simulink model "Path_following_Model_w_dbl_lane_change"  (R2018a)
settings: Solver=VariableStepAuto  StartTime=0.0  StopTime=inf  FixedStep=1  RelTol=1e-3
values from neighbouring files (symbols this model uses):
  A_matrix = [a11 a12 0 0; a21 a22 0 0; 0 1 0 0; V ls V 0]    [Path_following_SS.m]
  B_matrix = [b11 0; b21 0; 0 -V; 0 -ls*V]    [Path_following_SS.m]
  C_matrix = [1 0 0 0; 0 1 0 0; 0 0 1 0; 0 0 0 1]    [Path_following_SS.m]
  D_matrix = [0 0; 0 0; 0 0; 0 0]    [Path_following_SS.m]
  dis_vec = Cum_dis(1:end-1)    [Double_lane_change_bezier_func_mcode_V2.m]
  rho_new = (((del_1_Xp(2:end)/del_pts).*(del_2_Yp/del_pts.^2))-((del_1_Yp(2:end)/del_pts).*((del_2_Xp/del_pts.^2))))./((del_1_Xp(2:end)./del_pts).^2+((del_1_Yp(2:end)./del_pts).^2)).^1.5    [Double_lane_change_bezier_func_mcode_V2.m]
  V = 5    [Path_following_SS.m]
  Xp = [Xp_1(1:end-1); Xp_2(1:end-1); Xp_3(1:end-1);]    [Double_lane_change_bezier_func_mcode_V2.m]
  Yp = [Yp_1(1:end-1); Yp_2(1:end-1); Yp_3(1:end-1);]    [Double_lane_change_bezier_func_mcode_V2.m]
undefined symbols (not defined in the file or in its folder): Cum_dis, sigbuilder_block
libraries: simulink x2
settings Model: Creator=Santo  LastModifiedBy=SYG

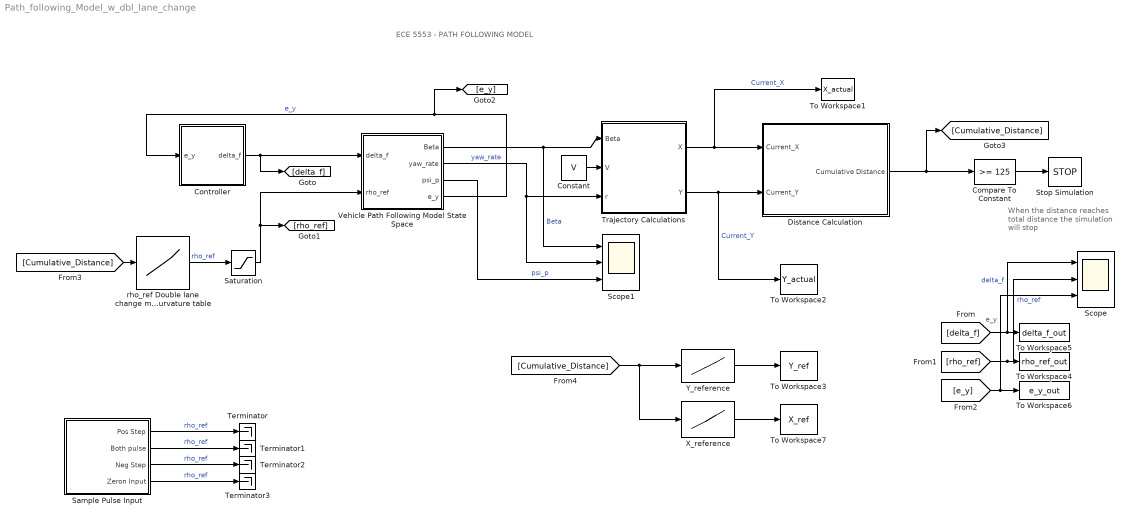
== system Path_following_Model_w_dbl_lane_change ==
  note: When the distance reaches total distance the simulation will stop
  note: ECE 5553 - PATH FOLLOWING MODEL
  Compare To Constant : simulink/Logic and Bit Operations/Compare To Constant  relop=>=  const=125  OutDataTypeStr=boolean
  Constant : Constant  Value=V
  Controller : Subsystem
  Distance Calculation : Subsystem
  Sample Pulse Input : Subsystem  Tag=STV Subsys  LoadFcn=sigbuilder_block('load');  StartFcn=sigbuilder_block('start');  StopFcn=sigbuilder_block('stop');  ClipboardFcn=sigbuilder_block('clipboard');  mask(Sigbuilder block){tuvar=[0:10]}
      mask help: Simulink:masks:SigbuilderBlock_MD
      mask init:
      | if ~strcmp(get_param(bdroot(gcbh),'SimulationStatus'),'stopped') tuvar = sigbuilder_block('maskInit'); end
      settings: CopyFcn=sigbuilder_block('copy');  DeleteFcn=sigbuilder_block('delete');  ModelCloseFcn=sigbuilder_block('modelClose');  PreSaveFcn=sigbuilder_block('preSave');  PauseFcn=sigbuilder_block('pause');  ContinueFcn=sigbuilder_block('continue');  NameChangeFcn=sigbuilder_block('namechange');  OpenFcn=sigbuilder_block('open',[6 24 1012.5 453.75 ]);  CloseFcn=sigbuilder_block('close');
      mask Display: plot(0, 0, 100, 100,[2, 2, 32, 32, 2], [68, 8, 8, 68, 68],[32, 2], [38, 38], [32, 19, 2],[53, 60, 44], [32, 17, 17, 2],[16, 16, 31, 31]);txt = getActiveGroup(gcbh);text(2, 100, txt,'verticalAlignment', 'top');
  Saturation : Saturate  UpperLimit=0.01  LowerLimit=-0.025  LinearizeAsGain=off
  Scope : Scope  NumInputPorts=3
  Scope1 : Scope  NumInputPorts=3
  Stop Simulation : Stop
  Terminator{,1..3} (4 alike) : Terminator
  To Workspace1 : ToWorkspace  VariableName=X_actual  SampleTime=-1
  To Workspace2 : ToWorkspace  VariableName=Y_actual  SampleTime=-1
  To Workspace3 : ToWorkspace  VariableName=Y_ref  SampleTime=-1
  To Workspace4 : ToWorkspace  VariableName=rho_ref_out  SampleTime=-1
  To Workspace5 : ToWorkspace  VariableName=delta_f_out  SampleTime=-1
  To Workspace6 : ToWorkspace  VariableName=e_y_out  SampleTime=-1
  To Workspace7 : ToWorkspace  VariableName=X_ref  SampleTime=-1
  Trajectory Calculations : Subsystem
  Vehicle Path Following Model State Space : Subsystem
  X_reference : Lookup_n-D  NumberOfTableDimensions=1  BreakpointsForDimension1=Cum_dis  Table=Xp(1:end-1)  InternalRulePriority=Speed  RndMeth=Simplest  InputSameDT=on
  Y_reference : Lookup_n-D  NumberOfTableDimensions=1  BreakpointsForDimension1=Cum_dis  Table=Yp(1:end-1)  InternalRulePriority=Speed  RndMeth=Simplest  InputSameDT=on
  rho_ref Double lane change manoeuver distanced based Road curvature table : Lookup_n-D  NumberOfTableDimensions=1  BreakpointsForDimension1=dis_vec  Table=rho_new  InternalRulePriority=Speed  RndMeth=Simplest  InputSameDT=on
  wires:
  Trajectory Calculations/1(X) -> Distance Calculation/1(Current_X), To Workspace1/1  "Current_X"
  Constant/1 -> Trajectory Calculations/2(V)
  Vehicle Path Following Model State Space/4(e_y) -> [e_y], Controller/1(e_y)  "e_y"
  Vehicle Path Following Model State Space/1(Beta) -> Scope1/1, Trajectory Calculations/1(Beta)  "Beta"
  Vehicle Path Following Model State Space/2(yaw_rate) -> Scope1/2, Trajectory Calculations/3(r)  "yaw_rate"
  Controller/1(delta_f) -> [delta_f], Vehicle Path Following Model State Space/1(delta_f)
  [delta_f] -> Scope/1, To Workspace5/1  "delta_f"
  [rho_ref] -> Scope/2, To Workspace4/1  "rho_ref"
  [e_y] -> Scope/3, To Workspace6/1  "e_y"
  Vehicle Path Following Model State Space/3(psi_p) -> Scope1/3  "psi_p"
  Trajectory Calculations/2(Y) -> To Workspace2/1, Distance Calculation/2("Current_Y ")  "Current_Y"
  rho_ref Double lane change manoeuver distanced based Road curvature table/1 -> Saturation/1  "rho_ref"
  Compare To Constant/1 -> Stop Simulation/1
  Saturation/1 -> Vehicle Path Following Model State Space/2(rho_ref), [rho_ref]
  Distance Calculation/1(Cumulative Distance) -> [Cumulative_Distance], Compare To Constant/1
  Sample Pulse Input/1(Pos Step) -> Terminator/1  "rho_ref"
  Sample Pulse Input/2(Both pulse) -> Terminator1/1  "rho_ref"
  Sample Pulse Input/3(Neg Step) -> Terminator2/1  "rho_ref"
  Sample Pulse Input/4(Zeron Input) -> Terminator3/1  "rho_ref"
  X_reference/1 -> To Workspace7/1
  Y_reference/1 -> To Workspace3/1
  [Cumulative_Distance] -> rho_ref Double lane change manoeuver distanced based Road curvature table/1
  [Cumulative_Distance] -> X_reference/1, Y_reference/1

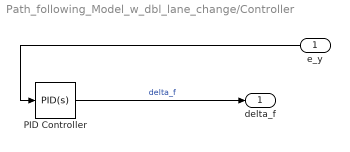
== system Path_following_Model_w_dbl_lane_change/Controller ==
  e_y : Inport
  PID Controller : simulink/Continuous/PID Controller  Controller=PID  TimeDomain=Continuous-time  SampleTime=-1  IntegratorMethod=Forward Euler  FilterMethod=Forward Euler  Form=Parallel  UseFilter=on  ControllerParametersSource=internal  P=-3.00951214129924  I=-3.08390402818753  D=0.0317765423784897  N=10.6234395055982  InitialConditionSource=internal  InitialConditionForIntegrator=0  InitialConditionForFilter=0  ExternalReset=none  LimitOutput=off  UpperSaturationLimit=inf  LowerSaturationLimit=-inf  LinearizeAsGain=on  AntiWindupMode=none  Kb=1  TrackingMode=off  Kt=1  PParamMin=[]  PParamMax=[]  IParamMin=[]  IParamMax=[]  DParamMin=[]  DParamMax=[]  NParamMin=[]  NParamMax=[]  KbParamMin=[]  KbParamMax=[]  KtParamMin=[]  KtParamMax=[]  POutMin=[]  POutMax=[]  IOutMin=[]  IOutMax=[]  DOutMin=[]  DOutMax=[]  NOutMin=[]  NOutMax=[]  KbOutMin=[]  KbOutMax=[]  KtOutMin=[]  KtOutMax=[]  IntegratorOutMin=[]  IntegratorOutMax=[]  FilterOutMin=[]  FilterOutMax=[]  SumOutMin=[]  SumOutMax=[]  SumI1OutMin=[]  SumI1OutMax=[]  SumI2OutMin=[]  SumI2OutMax=[]  SumI3OutMin=[]  SumI3OutMax=[]  SumDOutMin=[]  SumDOutMax=[]  SaturationOutMin=[]  SaturationOutMax=[]  IntegratorContinuousStateAttributes=''  IntegratorStateMustResolveToSignalObject=off  IntegratorRTWStateStorageClass=Auto  FilterContinuousStateAttributes=''  FilterStateMustResolveToSignalObject=off  FilterRTWStateStorageClass=Auto  DifferentiatorICPrevScaledInput=0  DifferentiatorOutMin=[]  DifferentiatorOutMax=[]  InitialConditionSetting=State (most efficient)  FilterDiffOutCoefMin=[]  FilterDiffOutCoefMax=[]  SumDenOutMin=[]  SumDenOutMax=[]  SumNumOutMin=[]  SumNumOutMax=[]  ReciprocalOutMin=[]  ReciprocalOutMax=[]  DivideOutMin=[]  DivideOutMax=[]  TunerSelectOption=Transfer Function Based (PID Tuner App)
  delta_f : Outport
  wires:
  PID Controller/1 -> delta_f/1  "delta_f"
  e_y/1 -> PID Controller/1

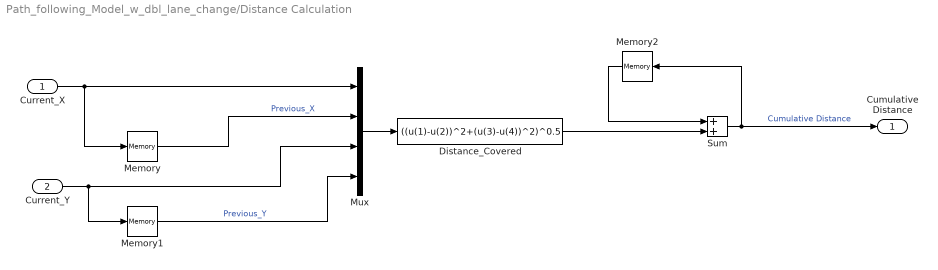
== system Path_following_Model_w_dbl_lane_change/Distance Calculation ==
  Current_X : Inport
  "Current_Y " : Inport  Port=2
  Distance_Covered : Fcn  Expr=((u(1)-u(2))^2+(u(3)-u(4))^2)^0.5
  Memory : Memory
  Memory1 : Memory
  Memory2 : Memory
  Mux : Mux
  Sum : Sum
  Cumulative Distance : Outport
  wires:
  Memory1/1 -> Mux/4  "Previous_Y"
  Mux/1 -> Distance_Covered/1
  Distance_Covered/1 -> Sum/2
  Memory/1 -> Mux/2  "Previous_X"
  Memory2/1 -> Sum/1
  "Current_Y "/1 -> Memory1/1, Mux/3
  Current_X/1 -> Memory/1, Mux/1
  Sum/1 -> Cumulative Distance/1, Memory2/1  "Cumulative Distance"

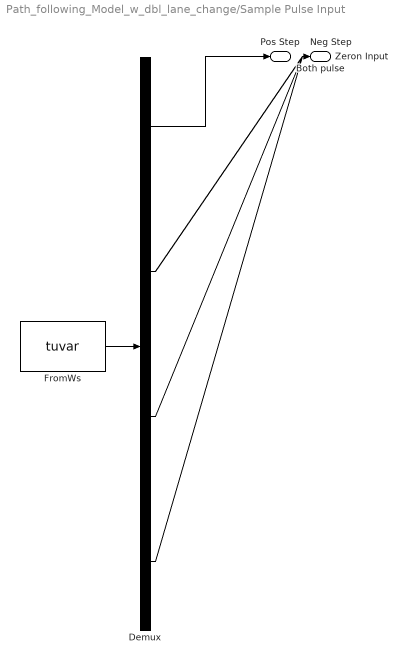
== system Path_following_Model_w_dbl_lane_change/Sample Pulse Input ==
  Demux : Demux  Tag=STV Demux
  FromWs : FromWorkspace  Tag=STV FromWs  VariableName=tuvar  SampleTime=0
      SigBuilderData=|
      | common.afterFinalStr = 'Extrapolate'
      | common.sampleTime = 0
      | dataSet.timeRange = [0 10]
      | dataSet.name = 'Group 1'
      | sbobj.Groups.Name = 'Group 1'
      | sbobj.Groups.Signals(1).Name = 'Pos Step'
      | sbobj.Groups.Signals(1).XData = [0 4 4 6 6 10]
      | sbobj.Groups.Signals(1).YData = [0 0 0.1 0.1 0 0]
      | sbobj.Groups.Signals(2).Name = 'Both pulse'
      | sbobj.Groups.Signals(2).XData = [0 4 4 6 6 7 7 9 9 10]
      | sbobj.Groups.Signals(2).YData = [0 0 0.1 0.1 0 0 -0.1 -0.1 0 0]
      | sbobj.Groups.Signals(3).Name = 'Neg Step'
      | sbobj.Groups.Signals(3).XData = [0 4 4 6 6 10]
      | sbobj.Groups.Signals(3).YData = [0 0 -0.1 -0.1 0 0]
      | sbobj.Groups.Signals(4).Name = 'Zeron Input'
      | sbobj.Groups.Signals(4).XData = [0 10]
      | sbobj.Groups.Signals(4).YData = [0 0]
  Pos Step : Outport  Tag=STV Outport
  Both pulse : Outport  Tag=STV Outport  Port=2
  Neg Step : Outport  Tag=STV Outport  Port=3
  Zeron Input : Outport  Tag=STV Outport  Port=4
  wires:
  FromWs/1 -> Demux/1
  Demux/1 -> Pos Step/1
  Demux/2 -> Both pulse/1
  Demux/3 -> Neg Step/1
  Demux/4 -> Zeron Input/1

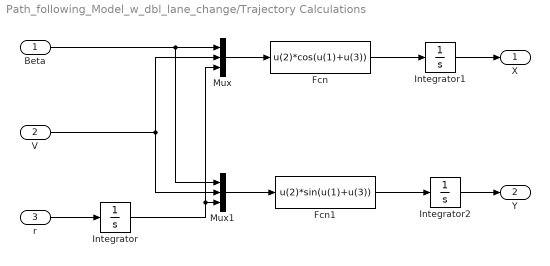
== system Path_following_Model_w_dbl_lane_change/Trajectory Calculations ==
  Beta : Inport
  V : Inport  Port=2
  r : Inport  Port=3
  Fcn : Fcn  Expr=u(2)*cos(u(1)+u(3))
  Fcn1 : Fcn  Expr=u(2)*sin(u(1)+u(3))
  Integrator : Integrator
  Integrator1 : Integrator  InitialCondition=Xp(1)
  Integrator2 : Integrator  InitialCondition=Yp(1)
  Mux : Mux  Inputs=3
  Mux1 : Mux  Inputs=3
  X : Outport
  Y : Outport  Port=2
  wires:
  Integrator2/1 -> Y/1
  Fcn1/1 -> Integrator2/1
  Integrator1/1 -> X/1
  Fcn/1 -> Integrator1/1
  Mux1/1 -> Fcn1/1
  Mux/1 -> Fcn/1
  Integrator/1 -> Mux1/3, Mux/3
  V/1 -> Mux1/2, Mux/2
  Beta/1 -> Mux1/1, Mux/1
  r/1 -> Integrator/1

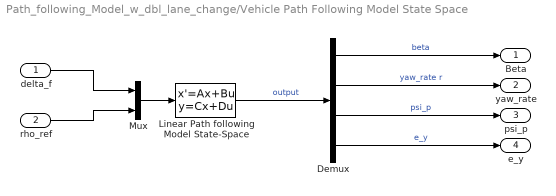
== system Path_following_Model_w_dbl_lane_change/Vehicle Path Following Model State Space ==
  delta_f : Inport
  rho_ref : Inport  Port=2
  Demux : Demux
  Linear Path following Model State-Space : StateSpace  A=A_matrix  B=B_matrix  C=C_matrix  D=D_matrix  InitialCondition=0
  Mux : Mux  Inputs=2
  Beta : Outport
  yaw_rate : Outport  Port=2
  psi_p : Outport  Port=3
  e_y : Outport  Port=4
  wires:
  Demux/4 -> e_y/1  "e_y"
  Mux/1 -> Linear Path following Model State-Space/1
  Demux/2 -> yaw_rate/1  "yaw_rate r"
  Linear Path following Model State-Space/1 -> Demux/1  "output"
  Demux/1 -> Beta/1  "beta"
  rho_ref/1 -> Mux/2
  delta_f/1 -> Mux/1
  Demux/3 -> psi_p/1  "psi_p"
